simulink model "ferment"  (Simulink 4.00)
settings: Solver=ode45  StartTime=0.0  StopTime=200  RelTol=1e-3
settings Model: LastModifiedBy=madarj  BlockReductionOpt=off

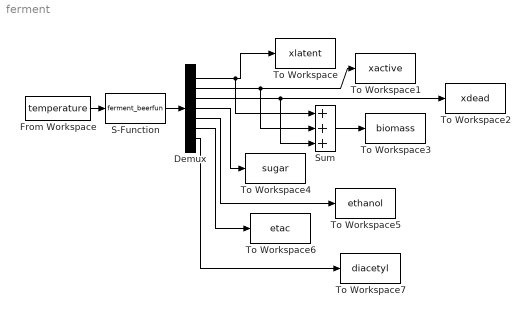
== system ferment ==
  Demux : Demux  Outputs=7  BusSelectionMode=off
  From Workspace : FromWorkspace  VariableName=temperature  SampleTime=0  OutputAfterFinalValue=Extrapolation
  S-Function : S-Function  FunctionName=ferment_beerfun  PortCounts=[]  SFunctionModules=''
  Sum : Sum  Inputs=+++  SaturateOnIntegerOverflow=off
  To Workspace : ToWorkspace  VariableName=xlatent  SampleTime=0  SaveFormat=Array
  To Workspace1 : ToWorkspace  VariableName=xactive  SampleTime=0  SaveFormat=Array
  To Workspace2 : ToWorkspace  VariableName=xdead  SampleTime=0  SaveFormat=Array
  To Workspace3 : ToWorkspace  VariableName=biomass  SampleTime=0  SaveFormat=Array
  To Workspace4 : ToWorkspace  VariableName=sugar  SampleTime=0  SaveFormat=Array
  To Workspace5 : ToWorkspace  VariableName=ethanol  SampleTime=0  SaveFormat=Array
  To Workspace6 : ToWorkspace  VariableName=etac  SampleTime=0  SaveFormat=Array
  To Workspace7 : ToWorkspace  VariableName=diacetyl  SampleTime=0  SaveFormat=Array
  wires:
  From Workspace/1 -> S-Function/1
  S-Function/1 -> Demux/1
  Demux/1 -> To Workspace/1, Sum/1
  Demux/2 -> To Workspace1/1, Sum/2
  Demux/3 -> To Workspace2/1, Sum/3
  Sum/1 -> To Workspace3/1
  Demux/4 -> To Workspace4/1
  Demux/5 -> To Workspace5/1
  Demux/6 -> To Workspace6/1
  Demux/7 -> To Workspace7/1
